simulink model "model_est_kalman"  (R2022a)
settings: Solver=ode23t  StartTime=0.0  StopTime=20  RelTol=1e-3
undefined symbols (not defined in the file or in its folder): A, B, betta, C, Const_input, D, GAMMA_0, theta
settings Model: Creator=asmax  LastModifiedBy=asmax

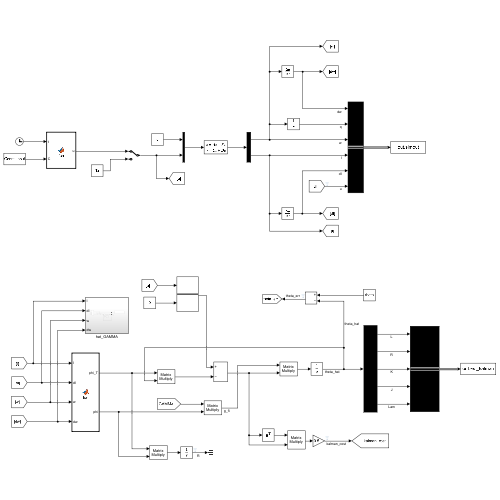
[thumbnail: Simulink's stored preview of the top-level diagram]
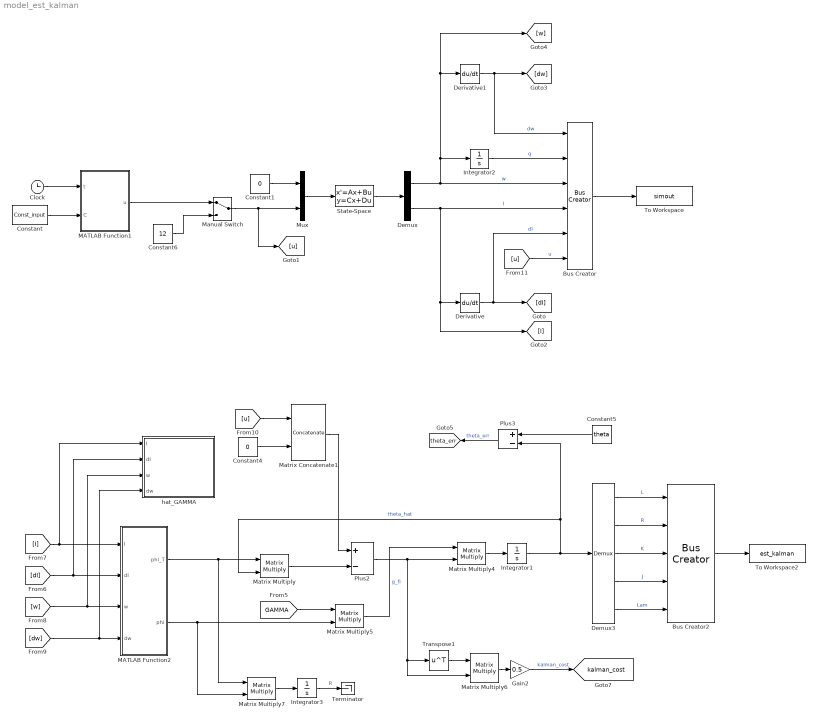
== system model_est_kalman ==
  Bus Creator : BusCreator  Inputs=6
  Bus Creator2 : BusCreator  Inputs=5
  Clock : Clock
  Constant : Constant  Value=Const_input
  Constant1 : Constant  Value=0
  Constant4 : Constant  Value=0
  Constant5 : Constant  Value=theta
  Constant6 : Constant  Value=12
  Demux : Demux  Outputs=2
  Demux3 : Demux  Outputs=5
  Derivative : Derivative
  Derivative1 : Derivative
  Gain2 : Gain  Gain=0.5
  Integrator1 : Integrator  InitialCondition=1
  Integrator2 : Integrator
  Integrator3 : Integrator
  MATLAB Function1 : MATLAB Function  TreatAsAtomicUnit=on
  MATLAB Function2 : MATLAB Function  TreatAsAtomicUnit=on
  Manual Switch : ManualSwitch
  Matrix Concatenate1 : Concatenate  ConcatenateDimension=2
  Matrix Multiply{,4..7} (5 alike) : Product  Multiplication=Matrix(*)
  Mux : Mux  Inputs=2
  Plus2 : Sum  Inputs=+-
  Plus3 : Sum  Inputs=+-
  State-Space : StateSpace  A=A  B=B  C=C  D=D  InitialCondition=[0;0]
  Terminator : Terminator
  To Workspace : ToWorkspace  VariableName=simout  SaveFormat=Timeseries  SampleTime=-1
  To Workspace2 : ToWorkspace  VariableName=est_kalman  SaveFormat=Timeseries  SampleTime=-1
  Transpose1 : Math  Operator=transpose
  hat_GAMMA : Subsystem
  tag scope: kalman_cost=global, theta_err=global
  wires:
  Mux/1 -> State-Space/1
  State-Space/1 -> Demux/1
  Constant1/1 -> Mux/1
  Demux/1 -> Integrator2/1, [w], Derivative1/1, Bus Creator/3  "w"
  Demux/2 -> [I], Derivative/1, Bus Creator/4  "I"
  Bus Creator/1 -> To Workspace/1
  Derivative/1 -> Bus Creator/5, [dI]  "dI"
  Derivative1/1 -> [dw], Bus Creator/1  "dw"
  Clock/1 -> MATLAB Function1/1(t)
  MATLAB Function2/1(phi_T) -> Matrix Multiply7/1, Matrix Multiply/1
  Matrix Multiply6/1 -> Gain2/1
  Transpose1/1 -> Matrix Multiply6/1
  MATLAB Function2/2(phi) -> Matrix Multiply7/2, Matrix Multiply5/2
  Gain2/1 -> [kalman_cost]  "kalman_cost"
  Matrix Concatenate1/1 -> Plus2/1
  Plus2/1 -> Matrix Multiply4/2, Matrix Multiply6/2, Transpose1/1
  Matrix Multiply/1 -> Plus2/2
  Matrix Multiply4/1 -> Integrator1/1
  [GAMMA] -> Matrix Multiply5/1
  Matrix Multiply5/1 -> Matrix Multiply4/1  "g_fi"
  [dI] -> MATLAB Function2/2(dI), hat_GAMMA/2(dI)
  [dw] -> hat_GAMMA/4(dw), MATLAB Function2/4(dw)
  [w] -> hat_GAMMA/3(w), MATLAB Function2/3(w)
  [I] -> hat_GAMMA/1(I), MATLAB Function2/1(I)
  Bus Creator2/1 -> To Workspace2/1
  Demux3/5 -> Bus Creator2/5  "Lam"
  Demux3/4 -> Bus Creator2/4  "J"
  Demux3/3 -> Bus Creator2/3  "K"
  Demux3/2 -> Bus Creator2/2  "R"
  Demux3/1 -> Bus Creator2/1  "L"
  [u] -> Matrix Concatenate1/1
  Constant4/1 -> Matrix Concatenate1/2
  Constant5/1 -> Plus3/1
  Integrator1/1 -> Demux3/1, Plus3/2, Matrix Multiply/2  "theta_hat"
  Plus3/1 -> [theta_err]  "theta_err"
  Manual Switch/1 -> [u], Mux/2
  MATLAB Function1/1(u) -> Manual Switch/1
  Constant6/1 -> Manual Switch/2
  Integrator2/1 -> Bus Creator/2  "q"
  [u] -> Bus Creator/6  "u"
  Matrix Multiply7/1 -> Integrator3/1
  Integrator3/1 -> Terminator/1  "R"
  Constant/1 -> MATLAB Function1/2(C)

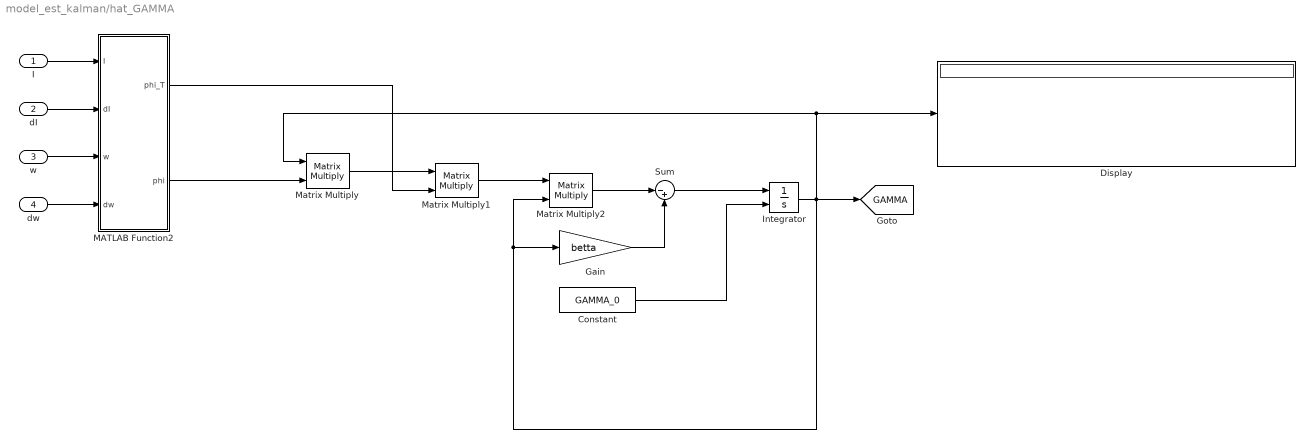
== system model_est_kalman/hat_GAMMA ==
  I : Inport
  dI : Inport  Port=2
  w : Inport  Port=3
  dw : Inport  Port=4
  Constant : Constant  Value=GAMMA_0
  Display : Display
  Gain : Gain  Gain=betta
  Integrator : Integrator  InitialConditionSource=external  InitialCondition=GAMMA_0
  MATLAB Function2 : MATLAB Function  TreatAsAtomicUnit=on
  Matrix Multiply : Product  Multiplication=Matrix(*)
  Matrix Multiply1 : Product  Multiplication=Matrix(*)
  Matrix Multiply2 : Product  Multiplication=Matrix(*)
  Sum : Sum  Inputs=|-+
  tag scope: GAMMA=global
  wires:
  Matrix Multiply/1 -> Matrix Multiply1/1
  Matrix Multiply1/1 -> Matrix Multiply2/1
  Matrix Multiply2/1 -> Sum/1
  Gain/1 -> Sum/2
  Sum/1 -> Integrator/1
  Integrator/1 -> Matrix Multiply/1, Display/1, [GAMMA], Matrix Multiply2/2, Gain/1
  MATLAB Function2/2(phi) -> Matrix Multiply/2
  MATLAB Function2/1(phi_T) -> Matrix Multiply1/2
  Constant/1 -> Integrator/2
  I/1 -> MATLAB Function2/1(I)
  w/1 -> MATLAB Function2/3(w)
  dI/1 -> MATLAB Function2/2(dI)
  dw/1 -> MATLAB Function2/4(dw)

== matlab function model_est_kalman/MATLAB Function2 ==
  data: phi_T output; phi output; I input; dI input; w input; dw input
function [phi_T, phi]= fcn(I, dI, w, dw)

phi = [dI 0;
     I 0;
     w -I;
     0 dw;
     0 w];
phi_T = phi';

== matlab function model_est_kalman/MATLAB Function1 ==
  data: t input; u output; C input
function u = fcn(t, C)

% matlab tests
% w = 6;
% A = 6;
% B = 6;
% fi = 3.1415;
% u = A * cos(w * t + fi) + B;

%real tests
% w = 1;
% A = 6;
% B = 6;
% fi = 3.1415;
% u = A * cos(w * t + fi) + B;

w = C(3);
A = C(1);
B = C(2);
fi = C(4);
u = A * cos(w * t + fi) + B;

== matlab function model_est_kalman/hat_GAMMA/MATLAB Function2 ==
  data: phi_T output; phi output; I input; dI input; w input; dw input
function [phi_T, phi]= fcn(I, dI, w, dw)

% phi = zeros(5,2);
% phi(1,1) = dI;
% phi(2,1) = I;
% phi(3,1) = w;
% phi(2,2) = ddq(1)*c2 + dq(1)^2*s2;
% 
% phi(3,2) = ddq(1);
% phi(4,2) = ddq(2);
% phi(5,1) = dq(1);
phi = [dI 0;
     I 0;
     w -I;
     0 dw;
     0 w];
phi_T = phi';
